simulink subsystem "calcErrorOuterLoop"  (R2026a)
settings: Solver=VariableStepAuto
settings Model: Creator=maxhu  LastModifiedBy=maxhu

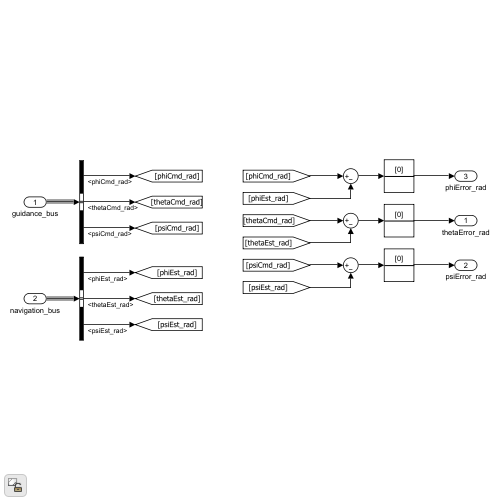
[thumbnail: Simulink's stored preview of the top-level diagram]
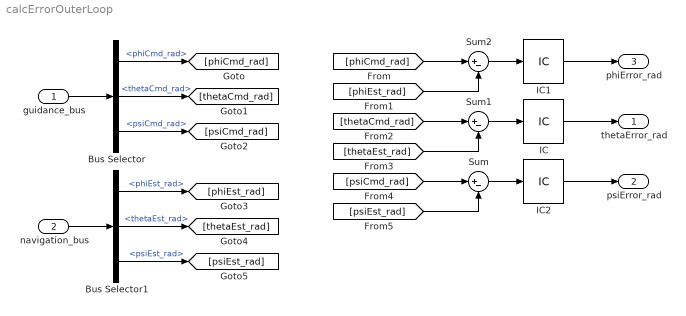
== system calcErrorOuterLoop ==
  guidance_bus : Inport
  navigation_bus : Inport  Port=2
  Bus Selector : BusSelector  OutputSignals=phiCmd_rad,thetaCmd_rad,psiCmd_rad
  Bus Selector1 : BusSelector  OutputSignals=phiEst_rad,thetaEst_rad,psiEst_rad
  IC : InitialCondition  Value=0
  IC1 : InitialCondition  Value=0
  IC2 : InitialCondition  Value=0
  Sum : Sum  Inputs=|+-
  Sum1 : Sum  Inputs=|+-
  Sum2 : Sum  Inputs=|+-
  thetaError_rad : Outport
  psiError_rad : Outport  Port=2
  phiError_rad : Outport  Port=3
  wires:
  [psiEst_rad] -> Sum/2
  guidance_bus/1 -> Bus Selector/1
  [thetaCmd_rad] -> Sum1/1
  navigation_bus/1 -> Bus Selector1/1
  Bus Selector1/1 -> [phiEst_rad]  "<phiEst_rad>"
  Bus Selector/2 -> [thetaCmd_rad]  "<thetaCmd_rad>"
  [phiCmd_rad] -> Sum2/1
  Bus Selector/1 -> [phiCmd_rad]  "<phiCmd_rad>"
  Bus Selector1/3 -> [psiEst_rad]  "<psiEst_rad>"
  [psiCmd_rad] -> Sum/1
  [phiEst_rad] -> Sum2/2
  Bus Selector1/2 -> [thetaEst_rad]  "<thetaEst_rad>"
  [thetaEst_rad] -> Sum1/2
  Bus Selector/3 -> [psiCmd_rad]  "<psiCmd_rad>"
  Sum2/1 -> IC1/1
  Sum1/1 -> IC/1
  Sum/1 -> IC2/1
  IC2/1 -> psiError_rad/1
  IC/1 -> thetaError_rad/1
  IC1/1 -> phiError_rad/1
